simulink model "with_target_ce"  (R2016b)
settings: Solver=VariableStepAuto  StartTime=0.0  StopTime=10.0  RelTol=1e-3
undefined symbols (not defined in the file or in its folder): physconst
libraries: phasedenvlib x7, phasedtxrxlib x7, dspinverses x4
settings Model: Creator=CHAITRA  LastModifiedBy=priya

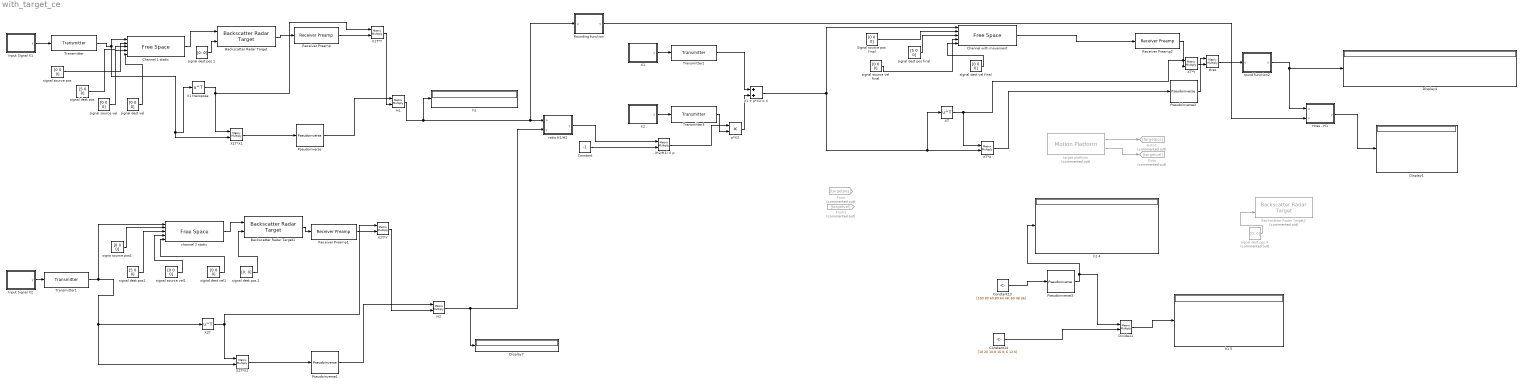
== system with_target_ce ==
  -(H2/H1) = p : Product  Multiplication=Matrix(*)
  Backscatter Radar Target : phasedenvlib/Backscatter Radar Target  EnablePolarization=off  AzimuthAngles=-180:180  ElevationAngles=-90:90  RCSPattern=ones(181,361)  ShhPattern=ones(181,361)  ShvPattern=ones(181,361)  SvvPattern=ones(181,361)  Model=Nonfluctuating  PropagationSpeed=physconst( 'LightSpeed' )  OperatingFrequency=3e8  SeedSource=Property  Seed=randi(65535,1)  SimulateUsing=Interpreted execution
  Backscatter Radar Target1 : phasedenvlib/Backscatter Radar Target  EnablePolarization=off  AzimuthAngles=-180:180  ElevationAngles=-90:90  RCSPattern=ones(181,361)  ShhPattern=ones(181,361)  ShvPattern=ones(181,361)  SvvPattern=ones(181,361)  Model=Nonfluctuating  PropagationSpeed=physconst( 'LightSpeed' )  OperatingFrequency=3e8  SeedSource=Property  Seed=randi(65535,1)  SimulateUsing=Interpreted execution
  Backscatter Radar Target2 : phasedenvlib/Backscatter Radar Target  Commented=on  EnablePolarization=off  AzimuthAngles=-180:180  ElevationAngles=-90:90  RCSPattern=ones(181,361)  ShhPattern=ones(181,361)  ShvPattern=ones(181,361)  SvvPattern=ones(181,361)  Model=Nonfluctuating  PropagationSpeed=physconst( 'LightSpeed' )  OperatingFrequency=3e8  SeedSource=Property  Seed=randi(65535,1)  SimulateUsing=Interpreted execution
  Channel 1 static : phasedenvlib/Free Space  PropagationSpeed=physconst( 'LightSpeed' )  OperatingFrequency=3e8  TwoWayPropagation=off  SampleRateFromInputCheckbox=off  SampleRate=100  MaximumDistanceSource=Property  MaximumDistance=10  MaximumNumInputSamplesSource=Auto  MaximumNumInputSamples=1000  SimulateUsing=Interpreted execution
  Channel with movement : phasedenvlib/Free Space  PropagationSpeed=physconst( 'LightSpeed' )  OperatingFrequency=3e8  TwoWayPropagation=off  SampleRateFromInputCheckbox=off  SampleRate=100  MaximumDistanceSource=Property  MaximumDistance=10  MaximumNumInputSamplesSource=Auto  MaximumNumInputSamples=1000  SimulateUsing=Interpreted execution
  Constant : Constant  Value=-1
  Constant13 : Constant  Value=[100 80 60;80 64 48; 60 48 36]
  Constant14 : Constant  Value=[10 20 10;8 16 8; 6 12 6]
  Display1 : Display
  Display4 : Display
  Display7 : Display
  Divide11 : Product  Multiplication=Matrix(*)
  From : From  Commented=on  GotoTag=targetpos
  From1 : From  Commented=on  GotoTag=targetvel
  Goto : Goto  Commented=on  GotoTag=targetvel
  Goto1 : Goto  Commented=on  GotoTag=targetpos
  H1 : Product  Multiplication=Matrix(*)
  H2 : Product  Multiplication=Matrix(*)
  Hres : Product  Multiplication=Matrix(*)
  Hres - H1 : MATLAB Function  TreatAsAtomicUnit=on
  Input Signal X1 : MATLAB Function  TreatAsAtomicUnit=on
  "Input Signal X2 " : MATLAB Function  TreatAsAtomicUnit=on
  Pseudoinverse{,1..3} (4 alike) : dspinverses/Pseudoinverse  wanterr=off  SimulateUsing=Interpreted execution
  Receiver Preamp : phasedtxrxlib/Receiver Preamp  Gain=20  LossFactor=0  NoiseMethod=Noise power  NoiseFigure=0  ReferenceTemperature=290  SampleRateFromInputCheckbox=on  SampleRate=1e6  NoisePower=0  EnableInputPort=off  PhaseNoiseInputPort=off  SeedSource=Property  Seed=randi(65535,1)  SimulateUsing=Interpreted execution
  Receiver Preamp1 : phasedtxrxlib/Receiver Preamp  Gain=20  LossFactor=0  NoiseMethod=Noise power  NoiseFigure=0  ReferenceTemperature=290  SampleRateFromInputCheckbox=on  SampleRate=1e6  NoisePower=0  EnableInputPort=off  PhaseNoiseInputPort=off  SeedSource=Property  Seed=randi(65535,1)  SimulateUsing=Interpreted execution
  Receiver Preamp2 : phasedtxrxlib/Receiver Preamp  Gain=20  LossFactor=0  NoiseMethod=Noise power  NoiseFigure=0  ReferenceTemperature=290  SampleRateFromInputCheckbox=on  SampleRate=1e6  NoisePower=0  EnableInputPort=off  PhaseNoiseInputPort=off  SeedSource=Property  Seed=randi(65535,1)  SimulateUsing=Interpreted execution
  Rounding function : MATLAB Function  TreatAsAtomicUnit=on
  Signal source pos final : Constant  Value=[0 0 0]
  Transmitter{,1..3} (4 alike) : phasedtxrxlib/Transmitter  PeakPower=5000  Gain=20  LossFactor=0  InUseOutputPort=off  CoherentOnTransmit=on  PhaseNoiseOutputPort=off  SeedSource=Property  Seed=randi(65535,1)  SimulateUsing=Interpreted execution
  X1 : MATLAB Function  TreatAsAtomicUnit=on
  X1 + p*X2 = X : Sum
  X1 transpose : Math  Operator=transpose  SaturateOnIntegerOverflow=on
  X1T*X1 : Product  Multiplication=Matrix(*)
  X1T*Y : Product  Multiplication=Matrix(*)
  X2 : MATLAB Function  TreatAsAtomicUnit=on
  X2T : Math  Operator=transpose  SaturateOnIntegerOverflow=on
  X2T*X2 : Product  Multiplication=Matrix(*)
  X2T*Y : Product  Multiplication=Matrix(*)
  XT : Math  Operator=transpose  SaturateOnIntegerOverflow=on
  XT*X : Product  Multiplication=Matrix(*)
  XT*Y : Product  Multiplication=Matrix(*)
  channel 2 static : phasedenvlib/Free Space  PropagationSpeed=physconst( 'LightSpeed' )  OperatingFrequency=3e8  TwoWayPropagation=off  SampleRateFromInputCheckbox=off  SampleRate=100  MaximumDistanceSource=Property  MaximumDistance=10  MaximumNumInputSamplesSource=Auto  MaximumNumInputSamples=1000  SimulateUsing=Interpreted execution
  "h1 " : Display
  h1 4 : Display
  h1 5 : Display
  p*X2 : Product
  ratio H1/H2 : MATLAB Function  TreatAsAtomicUnit=on
  round function2 : MATLAB Function  TreatAsAtomicUnit=on
  signa source pos1 : Constant  Value=[0 0 0]
  "signal dest pos " : Constant  Value=[5 0 0]
  signal dest pos 1 : Constant  Value=[0; 0]
  signal dest pos 2 : Constant  Value=[0; 0]
  signal dest pos 3 : Constant  Commented=on  Value=[0; 0]
  signal dest pos final : Constant  Value=[5 0 0]
  "signal dest pos1 " : Constant  Value=[5 0 0]
  signal dest vel : Constant  Value=[0 0 0]
  signal dest vel final : Constant  Value=[0 0 0]
  signal dest vel1 : Constant  Value=[0 0 0]
  signal source pos : Constant  Value=[0 0 0]
  signal source vel : Constant  Value=[0 0 0]
  signal source vel final : Constant  Value=[0 0 0]
  signal source vel1 : Constant  Value=[0 0 0]
  "target platform " : phasedenvlib/Motion Platform  Commented=on  MotionModel=Velocity  InitialPosition=[5;0;0]  InitialVelocity=[ 0; 0; 0 ]  VelocitySource=Property  Velocity=[0;0;0]  AccelerationSource=Property  Acceleration=[0;0;0]  InitialOrientationAxes=eye( 3 )  OrientationAxesOutputPort=off  ElapsedTimeSource=Auto  SampleRateFromInputCheckbox=on  SampleRate=1e6  SimulateUsing=Interpreted execution
  wires:
  X1 transpose/1 -> X1T*X1/1, X1T*Y/1
  X1T*X1/1 -> Pseudoinverse/1
  X1T*Y/1 -> H1/2
  ratio H1/H2/1(y) -> -(H2/H1) = p/1
  Input Signal X1/1(y) -> Transmitter/1
  Receiver Preamp/1 -> X1T*Y/2
  Pseudoinverse/1 -> H1/1
  X2T/1 -> X2T*Y/1, X2T*X2/1
  X2T*X2/1 -> Pseudoinverse1/1
  X2T*Y/1 -> H2/2
  "Input Signal X2 "/1(y) -> Transmitter1/1
  Receiver Preamp1/1 -> X2T*Y/2
  Pseudoinverse1/1 -> H2/1
  XT/1 -> XT*Y/1, XT*X/1
  XT*X/1 -> Pseudoinverse2/1
  XT*Y/1 -> Hres/2
  Receiver Preamp2/1 -> XT*Y/2
  Pseudoinverse2/1 -> Hres/1
  Constant/1 -> -(H2/H1) = p/2
  -(H2/H1) = p/1 -> p*X2/1
  X1/1(y) -> Transmitter2/1
  X2/1(y) -> Transmitter3/1
  Transmitter2/1 -> X1 + p*X2 = X/1
  Transmitter3/1 -> p*X2/2
  Transmitter/1 -> Channel 1 static/1, X1T*X1/2, X1 transpose/1
  Transmitter1/1 -> channel 2 static/1, X2T*X2/2, X2T/1
  H2/1 -> Display7/1, ratio H1/H2/2(v)
  X1 + p*X2 = X/1 -> XT*X/2, XT/1, Channel with movement/1
  p*X2/1 -> X1 + p*X2 = X/2
  signal source pos/1 -> Channel 1 static/2
  "signal dest pos "/1 -> Channel 1 static/3
  signal source vel/1 -> Channel 1 static/4
  signal dest vel/1 -> Channel 1 static/5
  signa source pos1/1 -> channel 2 static/2
  "signal dest pos1 "/1 -> channel 2 static/3
  signal source vel1/1 -> channel 2 static/4
  signal dest vel1/1 -> channel 2 static/5
  Signal source pos final/1 -> Channel with movement/2
  signal source vel final/1 -> Channel with movement/4
  signal dest vel final/1 -> Channel with movement/5
  Constant13/1 -> Pseudoinverse3/1
  Pseudoinverse3/1 -> Divide11/1, h1 4/1
  Constant14/1 -> Divide11/2
  Divide11/1 -> h1 5/1
  Hres - H1/1(y) -> Display1/1
  Hres/1 -> round function2/1(u)
  round function2/1(y) -> Hres - H1/1(u), Display4/1
  H1/1 -> "h1 "/1, Rounding function/1(u), ratio H1/H2/1(u)
  Rounding function/1(y) -> Hres - H1/2(v)
  Channel 1 static/1 -> Backscatter Radar Target/1
  Backscatter Radar Target/1 -> Receiver Preamp/1
  signal dest pos 1/1 -> Backscatter Radar Target/2
  signal dest pos 2/1 -> Backscatter Radar Target1/2
  Backscatter Radar Target1/1 -> Receiver Preamp1/1
  channel 2 static/1 -> Backscatter Radar Target1/1
  Channel with movement/1 -> Receiver Preamp2/1
  "target platform "/2 -> Goto/1
  "target platform "/1 -> Goto1/1
  signal dest pos final/1 -> Channel with movement/3
  ? -> Backscatter Radar Target2/1
  signal dest pos 3/1 -> Backscatter Radar Target2/2

== matlab function with_target_ce/X1 ==
  data: y output
function y = fcn()

f = 1;
t = 0:0.01:1;

a = 5*sin(2*pi*f*t);
y = transpose(a);

== matlab function with_target_ce/X2 ==
  data: y output
function y = fcn()

f = 5;
t = 0:0.01:1;

a = 5*sin(2*pi*f*t);

y = transpose(a);

== matlab function with_target_ce/Hres - H1 ==
  data: u input; y output; v input
function y = fcn(u,v)

%y = ldivide(w,z)
% you can divide each element by the same eleent of other row by
y= u-v ;

== matlab function with_target_ce/ratio H1//H2 ==
  data: u input; y output; v input
function y = fcn(u,v)

%y = ldivide(w,z)
% you can divide each element by the same eleent of other row by
y= u./v ;

== matlab function with_target_ce/Input Signal X1 ==
  data: y output
function y = fcn()

f = 1;
t = 0:0.01:1;

a = 5*sin(2*pi*f*t);
y = transpose(a);

== matlab function with_target_ce/Input Signal X2  ==
  data: y output
function y = fcn()

f =1;
t = 0:0.01:1;

a = 5*sin(2*pi*f*t);

y = transpose(a);

== matlab function with_target_ce/round function2 ==
  data: u input; y output
function y = fcn(u)

y = round(u*100000000)/100000000;

== matlab function with_target_ce/Rounding function ==
  data: u input; y output
function y = fcn(u)

y = round(u*100000000)/100000000;
